simulink model "controlpurepursuit"  (R2020b)
settings: Solver=VariableStepAuto  StartTime=0.0  StopTime=70  RelTol=1e-3
values from neighbouring files (symbols this model uses):
  L = vehicleDims.Length    [PRMDubins.m]    (also in RRTstar.m)
  ld = 1.8    [PRMDubins.m]    (also in RRTstar.m)
  xRef = refstates(:,1)    [PRMDubins.m]    (also in RRTstar.m)
  yRef = refstates(:,2)    [PRMDubins.m]    (also in RRTstar.m)
libraries: robotalgslib x1, autolibshared x1
settings Model: Creator=Akshath  LastModifiedBy=Akshath

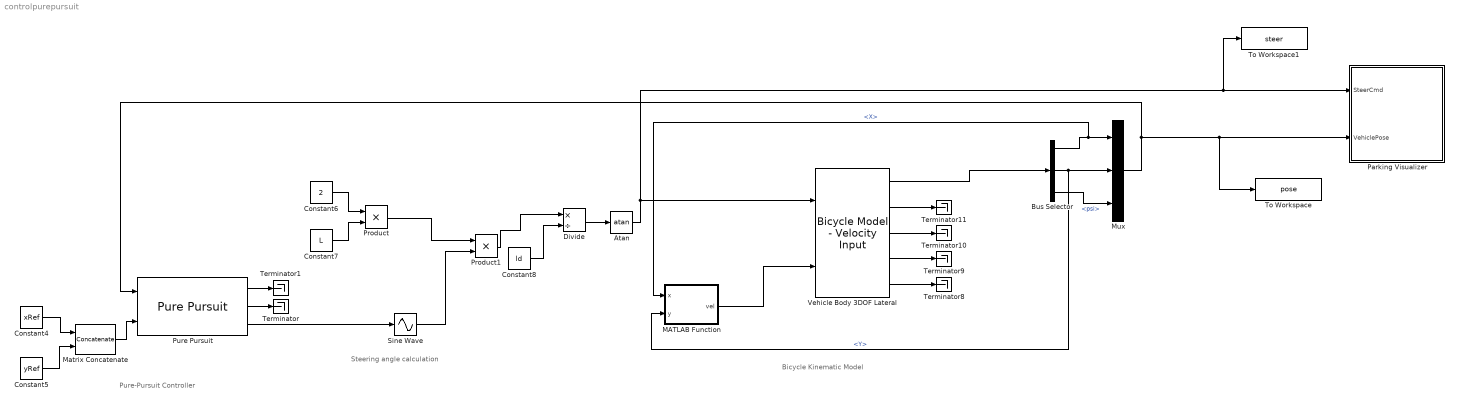
== system controlpurepursuit ==
  note: Bicycle Kinematic Model
  note: Pure-Pursuit Controller
  note: Steering angle calculation
  Atan : Trigonometry  Operator=atan
  Bus Selector : BusSelector  OutputSignals=InertFrm.Cg.Disp.X,InertFrm.Cg.Disp.Y,InertFrm.Cg.Ang.psi
  Constant4 : Constant  Value=xRef
  Constant5 : Constant  Value=yRef
  Constant6 : Constant  Value=2
  Constant7 : Constant  Value=L
  Constant8 : Constant  Value=ld
  Divide : Product  Inputs=*/
  MATLAB Function : MATLAB Function  TreatAsAtomicUnit=on
  Matrix Concatenate : Concatenate  Mode=Multidimensional array  ConcatenateDimension=2
  Mux : Mux  Inputs=3
  Parking Visualizer : Subsystem
  Product : Product
  Product1 : Product
  Pure Pursuit : robotalgslib/Pure Pursuit  DesiredLinearVelocity=0.1  MaxAngularVelocity=1.0  LookaheadDistance=ld  TargetDirPort=on  SimulateUsing=Code generation
  Sine Wave : Sin  TimeSource=Use external signal  SampleTime=0
  Terminator{,1,8..11} (6 alike) : Terminator
  To Workspace : ToWorkspace  VariableName=pose  SaveFormat=Timeseries  SampleTime=0.1
  To Workspace1 : ToWorkspace  VariableName=steer  SaveFormat=Timeseries  SampleTime=0.1
  Vehicle Body 3DOF Lateral : autolibshared/Bicycle Model - Velocity Input  trackMode=Single (bicycle)  inputMode=External longitudinal forces  frontSteerMode=on  rearSteerMode=off  windMode=off  muMode=off  extFMode=off  extMMode=off  aMode=3  NF=2  NR=2  m=2000  a=1.4  b=1.4  h=0.35  X_o=X_o  xdot_o=0  CalphaMode=off  sigmaMode=on  w=[1.4,1.4]  Cy_f=12e3  Cy_r=11e3  sigma_f=.1  sigma_r=.1  alpha_f_brk=[-.1 .1]  Cy_f_data=[-9e3 9e3]  alpha_r_brk=[-.1 .1]  Cy_r_data=[-9e3 9e3]  Y_o=Y_o  ydot_o=0  Izz=4000  psi_o=psi_o  r_o=0  Af=0  Cd=.3  Cl=.1  Cpm=.1  beta_w=[0:0.01:0.3]  Cs=[0:0.03:0.9]  Cym=[0:0.01:0.3]  Pabs=101325  Tair=273  g=9.81  mu=1  xdot_tol=0.01  Fznom=5000  Fxtire_sat=1e6  Fytire_sat=1e6  longOff=0  latOff=0  vertOff=0
      settings: SourceProductBaseCode=PW,MT,UV,VE,VP
  wires:
  Constant4/1 -> Matrix Concatenate/1
  Constant5/1 -> Matrix Concatenate/2
  Matrix Concatenate/1 -> Pure Pursuit/2
  Vehicle Body 3DOF Lateral/1 -> Bus Selector/1
  Bus Selector/1 -> MATLAB Function/1(x), Mux/1  "<X>"
  Bus Selector/2 -> Mux/2, MATLAB Function/2(y)  "<Y>"
  Bus Selector/3 -> Mux/3  "<psi>"
  Constant6/1 -> Product/1
  Constant7/1 -> Product/2
  Product/1 -> Product1/1
  Sine Wave/1 -> Product1/2
  Constant8/1 -> Divide/2
  Product1/1 -> Divide/1
  Divide/1 -> Atan/1
  Pure Pursuit/3 -> Sine Wave/1
  Atan/1 -> Parking Visualizer/1(SteerCmd), To Workspace1/1, Vehicle Body 3DOF Lateral/1
  Pure Pursuit/2 -> Terminator/1
  Mux/1 -> To Workspace/1, Parking Visualizer/2(VehiclePose), Pure Pursuit/1
  Vehicle Body 3DOF Lateral/5 -> Terminator8/1
  Vehicle Body 3DOF Lateral/4 -> Terminator9/1
  Vehicle Body 3DOF Lateral/2 -> Terminator11/1
  Vehicle Body 3DOF Lateral/3 -> Terminator10/1
  Pure Pursuit/1 -> Terminator1/1
  MATLAB Function/1(vel) -> Vehicle Body 3DOF Lateral/2

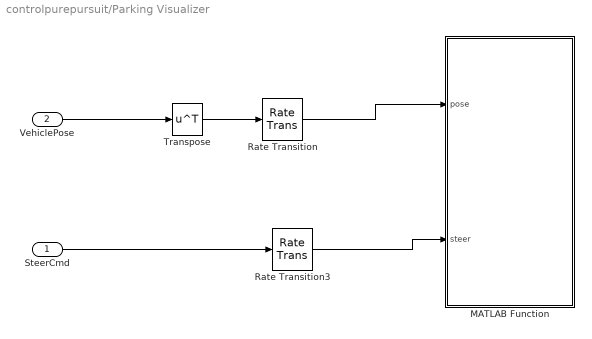
== system controlpurepursuit/Parking Visualizer ==
  SteerCmd : Inport
  VehiclePose : Inport  Port=2
  MATLAB Function : MATLAB Function  TreatAsAtomicUnit=on
  Rate Transition : RateTransition  Deterministic=off  OutPortSampleTime=Tv
  Rate Transition3 : RateTransition  Deterministic=off  OutPortSampleTime=Tv
  Transpose : Math  Operator=transpose  SaturateOnIntegerOverflow=on
  wires:
  Rate Transition3/1 -> MATLAB Function/2(steer)
  SteerCmd/1 -> Rate Transition3/1
  VehiclePose/1 -> Transpose/1
  Rate Transition/1 -> MATLAB Function/1(pose)
  Transpose/1 -> Rate Transition/1

== matlab function controlpurepursuit/MATLAB Function ==
  data: x input; vel output; y input
function vel = checkgoal(x,y)
% Function to check if the vehicle has reached the goal and setting the
% velocity to zero.
goal=[95.5, 38.5, pi/2];
dist = sqrt((x-goal(1))^2 + (y-goal(2))^2);
if dist<=1
    vel = 0;
else
    vel = 2;
end
end

== matlab function controlpurepursuit/Parking Visualizer/MATLAB Function ==
  data: pose input; steer input
function visualizeParking(pose, steer)

%visualizePath Display simulation results.

coder.extrinsic('VisualizeParking');

VisualizeParking(pose, steer);
end
